simulink model "Dynamic_Vibration_Absorber"  (R2024a)
settings: Solver=VariableStepAuto  StartTime=0.0  StopTime=10  MaxStep=0.001  RelTol=1e-3
model workspace (MAT data in the model file):
  b = 100
  k1 = 100
  k2 = 400
  m1 = 20
  m2 = 200
settings Model: Creator=91839
settings SolverCC: AlgebraicLoopSolver=TrustRegion
settings DataIOCC: ExternalInput=data  LoadExternalInput=on  SaveFormat=Array  DSMLogging=off  ReturnWorkspaceOutputs=off
settings DebuggingCC: UnconnectedInputMsg=warning  UnconnectedOutputMsg=warning  UnconnectedLineMsg=warning
settings ModelReferenceCC: EnableRefExpFcnMdlSchedulingChecks=on
settings SFSimCC: CustomCodeUndefinedFunction=UseInterfaceOnly
settings RTWCC: GPUComputeCapability=3.5

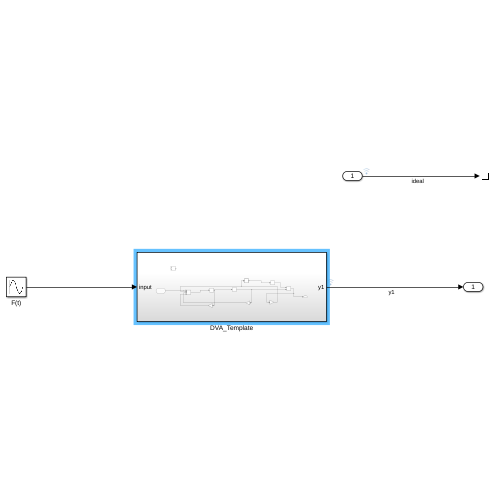
[thumbnail: Simulink's stored preview of the top-level diagram]
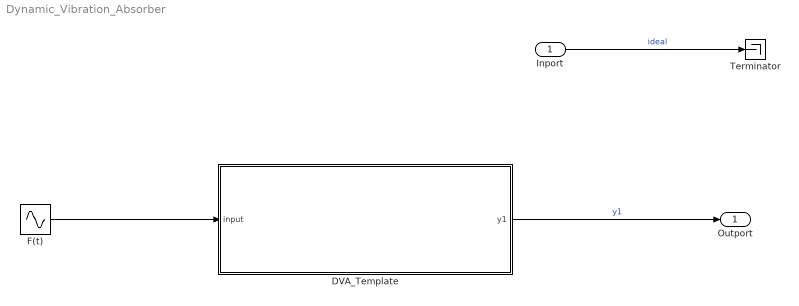
== system Dynamic_Vibration_Absorber ==
  Inport : Inport
  DVA_Template : Subsystem
  F(t) : Sin  Frequency=2  SampleTime=0
  Terminator : Terminator
  Outport : Outport
  wires:
  Inport/1 -> Terminator/1  "ideal"
  F(t)/1 -> DVA_Template/1(input)
  DVA_Template/1(y1) -> Outport/1  "y1"

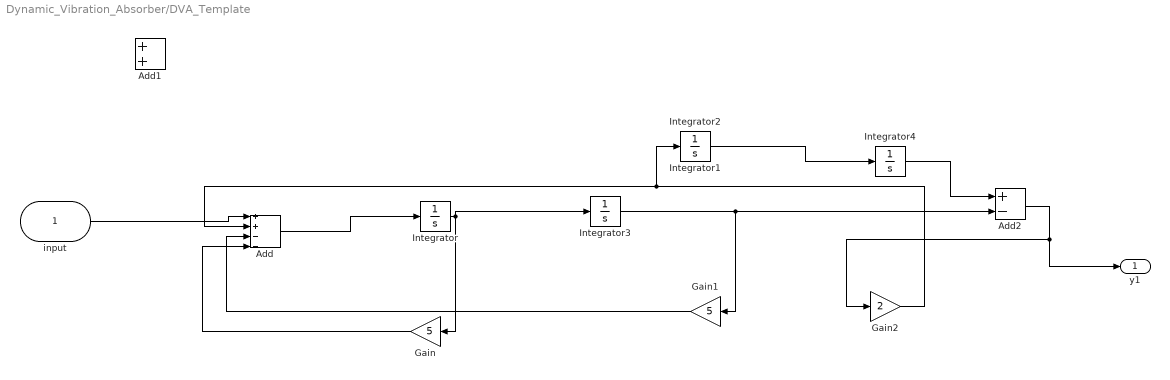
== system Dynamic_Vibration_Absorber/DVA_Template ==
  input : Inport
  Add : Sum  Inputs=++--
  Add1 : Sum
  Add2 : Sum  Inputs=+-
  Gain : Gain  Gain=5
  Gain1 : Gain  Gain=5
  Gain2 : Gain  Gain=2
  Integrator{,1..4} (5 alike) : Integrator
  y1 : Outport
  wires:
  input/1 -> Add/1
  Integrator/1 -> Gain/1, Integrator3/1
  Gain/1 -> Add/4
  Integrator3/1 -> Gain1/1, Add2/2
  Gain1/1 -> Add/3
  Add/1 -> Integrator/1
  Integrator2/1 -> Integrator4/1
  Integrator4/1 -> Add2/1
  Add2/1 -> y1/1, Gain2/1
  Gain2/1 -> Add/2, Integrator2/1
